simulink model "V2X_UDP_SCLX_Control_2019b"  (R2019b)
settings: Solver=FixedStepDiscrete  StartTime=0.0  StopTime=Inf  FixedStep=0.01  RelTol=1e-3
PostLoadFcn:
  | if any(exist('dsrtsu_mdlpostloadfcn', 'file') ~= 0), dsrtsu_mdlpostloadfcn('Execute', bdroot); end
InitFcn:
  | , if any(exist('rtifpga_mdlclblib', 'file') ~= 0), rtifpga_mdlclblib('Init', bdroot); end,
  | , if any(exist('dsmpb_private', 'file') ~= 0), dsmpb_private('dsmpb_mdlclblib', 'Init', bdroot); end,
values from neighbouring files (symbols this model uses):
  CtrlZone_Length = 250    [HDVPSG_DelayComp_NewRef_RealDrop_script_case1.m]
  High_TRFC = 1    [HDVPSG_DelayComp_NewRef_RealDrop_script_case1.m]
  PSG_AMAX = 3.2    [HDVPSG_DelayComp_NewRef_RealDrop_script_case1.m]
  PSG_AMIN = -6    [HDVPSG_DelayComp_NewRef_RealDrop_script_case1.m]
  PSG_first_v0 = 13    [HDVPSG_DelayComp_NewRef_RealDrop_script_case1.m]
  PSG_HighMu_D = 15    [HDVPSG_DelayComp_NewRef_RealDrop_script_case1.m]
  PSG_HighMu_I = 125    [HDVPSG_DelayComp_NewRef_RealDrop_script_case1.m]
  PSG_HighMu_P = 75    [HDVPSG_DelayComp_NewRef_RealDrop_script_case1.m]
  PSG_HighMu_TRFC = 0.8    [HDVPSG_DelayComp_NewRef_RealDrop_script_case1.m]
  PSG_LowMu_D = 12    [HDVPSG_DelayComp_NewRef_RealDrop_script_case1.m]
  PSG_LowMu_I = 64    [HDVPSG_DelayComp_NewRef_RealDrop_script_case1.m]
  PSG_LowMu_P = 48    [HDVPSG_DelayComp_NewRef_RealDrop_script_case1.m]
  PSG_LowMu_TRFC = 0.7    [HDVPSG_DelayComp_NewRef_RealDrop_script_case1.m]
  Q_Leader = 1    [HDVPSG_DelayComp_NewRef_RealDrop_script_case1.m]
  R_Leader = 20    [HDVPSG_DelayComp_NewRef_RealDrop_script_case1.m]
  T_ADE = 0.01    [HDVPSG_DelayComp_NewRef_RealDrop_script_case1.m]
  V_MAX = 40    [HDVPSG_DelayComp_NewRef_RealDrop_script_case1.m]
  V_MIN = 0    [HDVPSG_DelayComp_NewRef_RealDrop_script_case1.m]
undefined symbols (not defined in the file or in its folder): BETA_PSG_Leader, DiscIntNeverNeededParam, UT
libraries: simulink x4, dsmpblib x3
(part 3 of 3)

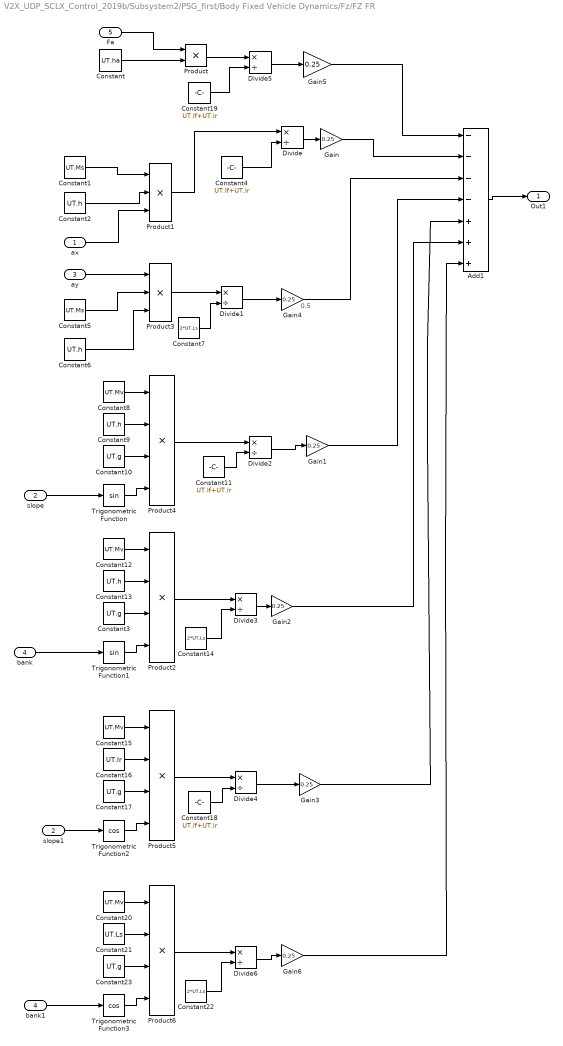
== system V2X_UDP_SCLX_Control_2019b/Subsystem2/PSG_first/Body Fixed Vehicle Dynamics/Fz/FZ FR ==
  note: 0.5
  ax : Inport
  slope : Inport  Port=2
  ay : Inport  Port=3
  bank : Inport  Port=4
  Fa : Inport  Port=5
  Add1 : Sum  Inputs=----+++
  Constant : Constant  Value=UT.ha
  Constant1 : Constant  Value=UT.Ms
  Constant{3,10,17,23} (4 alike) : Constant  Value=UT.g
  Constant{4,11,18..19} (4 alike) : Constant  Value=UT.lf+UT.lr
  Constant{8,12,15,20} (4 alike) : Constant  Value=UT.Mv
  Constant{2,6,9,13} (4 alike) : Constant  Value=UT.h
  Constant14 : Constant  Value=2*UT.Ls
  Constant16 : Constant  Value=UT.lr
  Constant21 : Constant  Value=UT.Ls
  Constant22 : Constant  Value=2*UT.Ls
  Constant5 : Constant  Value=UT.Ms
  Constant7 : Constant  Value=2*UT.Ls
  Divide{,1..6} (7 alike) : Product  Inputs=*/
  Gain{,1..6} (7 alike) : Gain  Gain=0.25
  Product : Product
  Product1 : Product  Inputs=3
  Product{2,4..6} (4 alike) : Product  Inputs=4
  Product3 : Product  Inputs=3
  Trigonometric Function : Trigonometry
  Trigonometric Function1 : Trigonometry
  Trigonometric Function2 : Trigonometry  Operator=cos
  Trigonometric Function3 : Trigonometry  Operator=cos
  bank1 : InportShadow  Port=4
  slope1 : InportShadow  Port=2
  Out1 : Outport  VectorParamsAs1DForOutWhenUnconnected=off
  wires:
  Gain6/1 -> Add1/7
  Divide6/1 -> Gain6/1
  Constant22/1 -> Divide6/2
  Product6/1 -> Divide6/1
  Trigonometric Function3/1 -> Product6/4
  bank1/1 -> Trigonometric Function3/1
  Constant23/1 -> Product6/3
  Constant21/1 -> Product6/2
  Constant20/1 -> Product6/1
  Gain2/1 -> Add1/6
  Gain4/1 -> Add1/3
  Gain3/1 -> Add1/5
  Gain1/1 -> Add1/4
  Gain/1 -> Add1/2
  Gain5/1 -> Add1/1
  Divide5/1 -> Gain5/1
  Constant19/1 -> Divide5/2
  Product/1 -> Divide5/1
  Constant/1 -> Product/2
  Fa/1 -> Product/1
  Product1/1 -> Divide/1
  Add1/1 -> Out1/1
  Divide4/1 -> Gain3/1
  Product5/1 -> Divide4/1
  Constant18/1 -> Divide4/2
  slope1/1 -> Trigonometric Function2/1
  Trigonometric Function2/1 -> Product5/4
  Constant17/1 -> Product5/3
  Constant16/1 -> Product5/2
  Constant15/1 -> Product5/1
  Divide3/1 -> Gain2/1
  Constant14/1 -> Divide3/2
  Product2/1 -> Divide3/1
  Trigonometric Function1/1 -> Product2/4
  bank/1 -> Trigonometric Function1/1
  Constant3/1 -> Product2/3
  Constant13/1 -> Product2/2
  Constant12/1 -> Product2/1
  Product4/1 -> Divide2/1
  Divide2/1 -> Gain1/1
  Constant11/1 -> Divide2/2
  Trigonometric Function/1 -> Product4/4
  slope/1 -> Trigonometric Function/1
  Constant10/1 -> Product4/3
  Constant9/1 -> Product4/2
  Constant8/1 -> Product4/1
  Divide1/1 -> Gain4/1
  Divide/1 -> Gain/1
  Constant7/1 -> Divide1/2
  Product3/1 -> Divide1/1
  Constant6/1 -> Product3/3
  Constant5/1 -> Product3/2
  ay/1 -> Product3/1
  Constant4/1 -> Divide/2
  ax/1 -> Product1/3
  Constant2/1 -> Product1/2
  Constant1/1 -> Product1/1

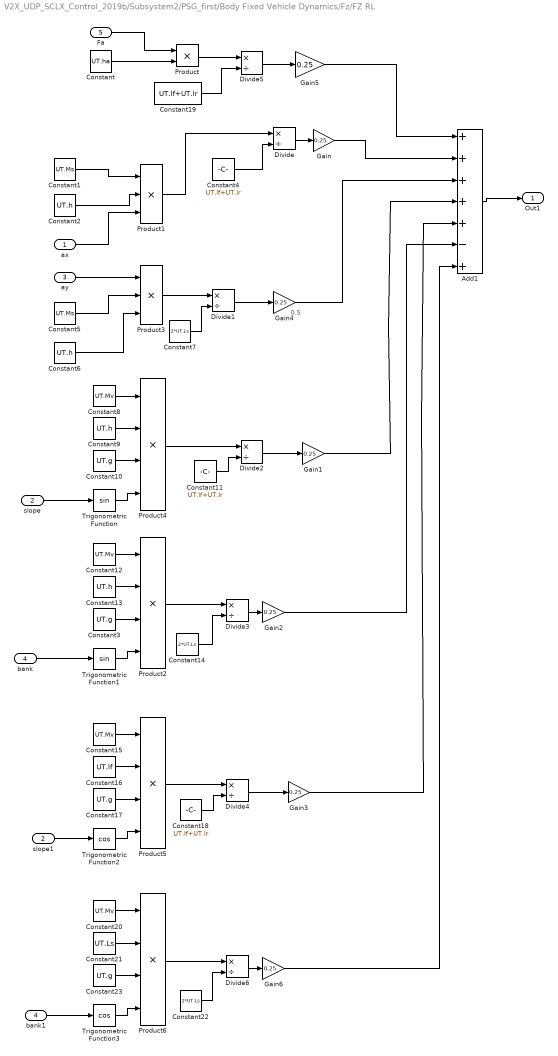
== system V2X_UDP_SCLX_Control_2019b/Subsystem2/PSG_first/Body Fixed Vehicle Dynamics/Fz/FZ RL ==
  note: 0.5
  ax : Inport
  slope : Inport  Port=2
  ay : Inport  Port=3
  bank : Inport  Port=4
  Fa : Inport  Port=5
  Add1 : Sum  Inputs=+++++-+
  Constant : Constant  Value=UT.ha
  Constant1 : Constant  Value=UT.Ms
  Constant{3,10,17,23} (4 alike) : Constant  Value=UT.g
  Constant{4,11,18..19} (4 alike) : Constant  Value=UT.lf+UT.lr
  Constant{8,12,15,20} (4 alike) : Constant  Value=UT.Mv
  Constant{2,6,9,13} (4 alike) : Constant  Value=UT.h
  Constant14 : Constant  Value=2*UT.Ls
  Constant16 : Constant  Value=UT.lf
  Constant21 : Constant  Value=UT.Ls
  Constant22 : Constant  Value=2*UT.Ls
  Constant5 : Constant  Value=UT.Ms
  Constant7 : Constant  Value=2*UT.Ls
  Divide{,1..6} (7 alike) : Product  Inputs=*/
  Gain{,1..6} (7 alike) : Gain  Gain=0.25
  Product : Product
  Product1 : Product  Inputs=3
  Product{2,4..6} (4 alike) : Product  Inputs=4
  Product3 : Product  Inputs=3
  Trigonometric Function : Trigonometry
  Trigonometric Function1 : Trigonometry
  Trigonometric Function2 : Trigonometry  Operator=cos
  Trigonometric Function3 : Trigonometry  Operator=cos
  bank1 : InportShadow  Port=4
  slope1 : InportShadow  Port=2
  Out1 : Outport  VectorParamsAs1DForOutWhenUnconnected=off
  wires:
  Gain6/1 -> Add1/7
  Divide6/1 -> Gain6/1
  Constant22/1 -> Divide6/2
  Product6/1 -> Divide6/1
  Trigonometric Function3/1 -> Product6/4
  bank1/1 -> Trigonometric Function3/1
  Constant23/1 -> Product6/3
  Constant21/1 -> Product6/2
  Constant20/1 -> Product6/1
  Gain2/1 -> Add1/6
  Gain4/1 -> Add1/3
  Gain3/1 -> Add1/5
  Gain1/1 -> Add1/4
  Gain/1 -> Add1/2
  Gain5/1 -> Add1/1
  Divide5/1 -> Gain5/1
  Constant19/1 -> Divide5/2
  Product/1 -> Divide5/1
  Constant/1 -> Product/2
  Fa/1 -> Product/1
  Product1/1 -> Divide/1
  Add1/1 -> Out1/1
  Divide4/1 -> Gain3/1
  Product5/1 -> Divide4/1
  Constant18/1 -> Divide4/2
  slope1/1 -> Trigonometric Function2/1
  Trigonometric Function2/1 -> Product5/4
  Constant17/1 -> Product5/3
  Constant16/1 -> Product5/2
  Constant15/1 -> Product5/1
  Divide3/1 -> Gain2/1
  Constant14/1 -> Divide3/2
  Product2/1 -> Divide3/1
  Trigonometric Function1/1 -> Product2/4
  bank/1 -> Trigonometric Function1/1
  Constant3/1 -> Product2/3
  Constant13/1 -> Product2/2
  Constant12/1 -> Product2/1
  Product4/1 -> Divide2/1
  Divide2/1 -> Gain1/1
  Constant11/1 -> Divide2/2
  Trigonometric Function/1 -> Product4/4
  slope/1 -> Trigonometric Function/1
  Constant10/1 -> Product4/3
  Constant9/1 -> Product4/2
  Constant8/1 -> Product4/1
  Divide1/1 -> Gain4/1
  Divide/1 -> Gain/1
  Constant7/1 -> Divide1/2
  Product3/1 -> Divide1/1
  Constant6/1 -> Product3/3
  Constant5/1 -> Product3/2
  ay/1 -> Product3/1
  Constant4/1 -> Divide/2
  ax/1 -> Product1/3
  Constant2/1 -> Product1/2
  Constant1/1 -> Product1/1

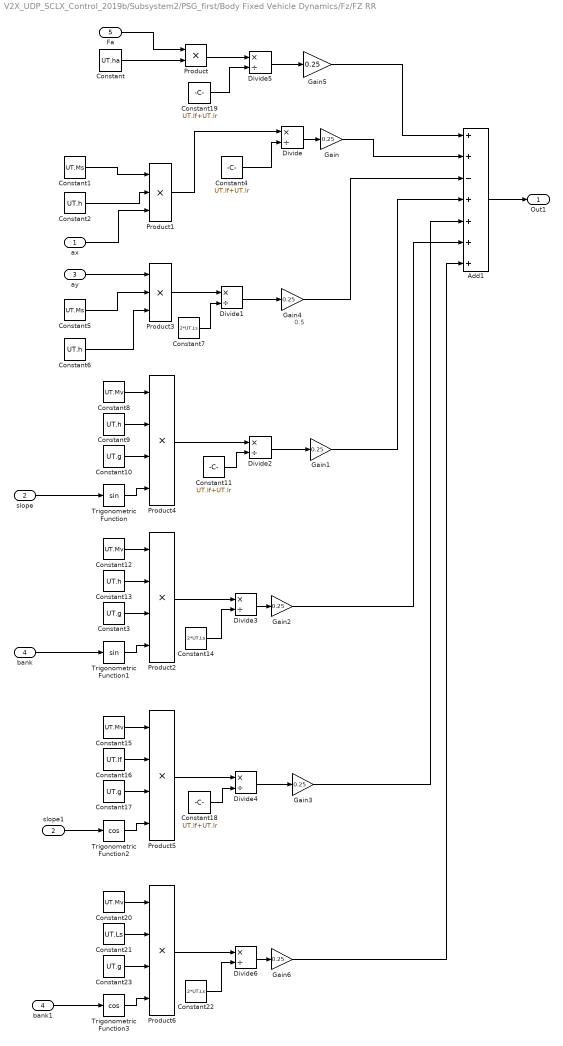
== system V2X_UDP_SCLX_Control_2019b/Subsystem2/PSG_first/Body Fixed Vehicle Dynamics/Fz/FZ RR ==
  note: 0.5
  ax : Inport
  slope : Inport  Port=2
  ay : Inport  Port=3
  bank : Inport  Port=4
  Fa : Inport  Port=5
  Add1 : Sum  Inputs=++-++++
  Constant : Constant  Value=UT.ha
  Constant1 : Constant  Value=UT.Ms
  Constant{3,10,17,23} (4 alike) : Constant  Value=UT.g
  Constant{4,11,18..19} (4 alike) : Constant  Value=UT.lf+UT.lr
  Constant{8,12,15,20} (4 alike) : Constant  Value=UT.Mv
  Constant{2,6,9,13} (4 alike) : Constant  Value=UT.h
  Constant14 : Constant  Value=2*UT.Ls
  Constant16 : Constant  Value=UT.lf
  Constant21 : Constant  Value=UT.Ls
  Constant22 : Constant  Value=2*UT.Ls
  Constant5 : Constant  Value=UT.Ms
  Constant7 : Constant  Value=2*UT.Ls
  Divide{,1..6} (7 alike) : Product  Inputs=*/
  Gain{,1..6} (7 alike) : Gain  Gain=0.25
  Product : Product
  Product1 : Product  Inputs=3
  Product{2,4..6} (4 alike) : Product  Inputs=4
  Product3 : Product  Inputs=3
  Trigonometric Function : Trigonometry
  Trigonometric Function1 : Trigonometry
  Trigonometric Function2 : Trigonometry  Operator=cos
  Trigonometric Function3 : Trigonometry  Operator=cos
  bank1 : InportShadow  Port=4
  slope1 : InportShadow  Port=2
  Out1 : Outport  VectorParamsAs1DForOutWhenUnconnected=off
  wires:
  Constant1/1 -> Product1/1
  Constant2/1 -> Product1/2
  ax/1 -> Product1/3
  Constant4/1 -> Divide/2
  ay/1 -> Product3/1
  Constant5/1 -> Product3/2
  Constant6/1 -> Product3/3
  Product3/1 -> Divide1/1
  Constant7/1 -> Divide1/2
  Divide/1 -> Gain/1
  Divide1/1 -> Gain4/1
  Constant8/1 -> Product4/1
  Constant9/1 -> Product4/2
  Constant10/1 -> Product4/3
  slope/1 -> Trigonometric Function/1
  Trigonometric Function/1 -> Product4/4
  Constant11/1 -> Divide2/2
  Divide2/1 -> Gain1/1
  Product4/1 -> Divide2/1
  Constant12/1 -> Product2/1
  Constant13/1 -> Product2/2
  Constant3/1 -> Product2/3
  bank/1 -> Trigonometric Function1/1
  Trigonometric Function1/1 -> Product2/4
  Product2/1 -> Divide3/1
  Constant14/1 -> Divide3/2
  Divide3/1 -> Gain2/1
  Constant15/1 -> Product5/1
  Constant16/1 -> Product5/2
  Constant17/1 -> Product5/3
  Trigonometric Function2/1 -> Product5/4
  slope1/1 -> Trigonometric Function2/1
  Constant18/1 -> Divide4/2
  Product5/1 -> Divide4/1
  Divide4/1 -> Gain3/1
  Add1/1 -> Out1/1
  Product1/1 -> Divide/1
  Fa/1 -> Product/1
  Constant/1 -> Product/2
  Product/1 -> Divide5/1
  Constant19/1 -> Divide5/2
  Divide5/1 -> Gain5/1
  Gain5/1 -> Add1/1
  Gain/1 -> Add1/2
  Gain1/1 -> Add1/4
  Gain3/1 -> Add1/5
  Gain4/1 -> Add1/3
  Gain2/1 -> Add1/6
  Constant20/1 -> Product6/1
  Constant21/1 -> Product6/2
  Constant23/1 -> Product6/3
  bank1/1 -> Trigonometric Function3/1
  Trigonometric Function3/1 -> Product6/4
  Product6/1 -> Divide6/1
  Constant22/1 -> Divide6/2
  Divide6/1 -> Gain6/1
  Gain6/1 -> Add1/7

== matlab function V2X_UDP_SCLX_Control_2019b/Double2Bytes1/MATLAB Function3 ==
  data: defloatMe input; byte1 output; byte2 output; byte3 output; byte4 output
function [byte1, byte2, byte3, byte4] = defloater(defloatMe)

% This block converts a single floating point number into a 4 byte vector
% based on IEEE-754 standard. By default, byte order is for little endian
% format - use the fliplr function to send big endian.

%float32 = zeros(1, 1, 'single');
float32 = typecast(single(defloatMe), 'uint8');
float32 = fliplr(float32);
byte1 = float32(1);
byte2 = float32(2);
byte3 = float32(3);
byte4 = float32(4);

== matlab function V2X_UDP_SCLX_Control_2019b/Bytes2Double/MATLAB Function2 ==
  data: byte1 input; float32 output; byte2 input; byte3 input; byte4 input
function float32 = floater(byte1, byte2, byte3, byte4)

% This block converts 4 uint8 values into a single floating point number
% based on IEEE-754 standard. By default, byte order is for little endian
% format - use the fliplr function to read big endian.

bytes = zeros(1, 4, 'uint8');
bytes = uint8([byte1, byte2, byte3, byte4]);
bytes = fliplr(bytes);
float32 = zeros(1, 1, 'single');
float32 = typecast(bytes,'single');

== matlab function V2X_UDP_SCLX_Control_2019b/MATLAB Function ==
  data: v_ref input; vref_vec output size=[21,1]
function vref_vec = fcn(v_ref)
   vref_vec = ones(21,1)*v_ref;
end

== matlab function V2X_UDP_SCLX_Control_2019b/Bytes2Double2/MATLAB Function2 ==
  data: byte1 input; float32 output; byte2 input; byte3 input; byte4 input
function float32 = floater(byte1, byte2, byte3, byte4)

% This block converts 4 uint8 values into a single floating point number
% based on IEEE-754 standard. By default, byte order is for little endian
% format - use the fliplr function to read big endian.

bytes = zeros(1, 4, 'uint8');
bytes = uint8([byte1, byte2, byte3, byte4]);
bytes = fliplr(bytes);
float32 = zeros(1, 1, 'single');
float32 = typecast(bytes,'single');

== matlab function V2X_UDP_SCLX_Control_2019b/ARE_First_Order_Derivative_[1,0,0]6/MATLAB Function ==
  data: U input; Dot_U output; Ts input; u_init input
function Dot_U = buffer(U, Ts, u_init)
    N = 12;
    %Ts = 0.01;
    persistent y;
    if isempty(y)
        y=u_init*ones(N+1,1);%m/s
    end

    y = [U;y(1:end-1)];
    T = Ts*N;
    P = zeros(1,N+1);
    P_alpha = P;
    for k = 1:N+1
        tao_k = (k-1)*Ts;
        P(k) = T-2*tao_k;
        if((k==1)||(k==N+1))
            P_alpha(k) = P(k)*Ts/2;
        else
            P_alpha(k) = P(k)*Ts;
        end
    end
    
    Dot_U = P_alpha*y*6/(T^3);

end

== matlab function V2X_UDP_SCLX_Control_2019b/leader_ulmpc_spd_ctrl/Sys_Leader ==
  data: Ts input; A output; B output; dk output; beta input; v_dot_hat input
function [A,B,dk] = f(Ts, beta, v_dot_hat)
    A  = 1;
    B  = beta*Ts;
    dk = v_dot_hat*Ts;
end
